simulink model "Acceleration_Angular__Spectrum_Analyser"  (R2014a)
settings: Solver=ode45  StartTime=0.0  StopTime=inf  RelTol=1e-3
undefined symbols (not defined in the file): NULL, serial
libraries: instrumentlib x2
settings Model: Creator=ddtdanilo  LastModifiedBy=ddtdanilo

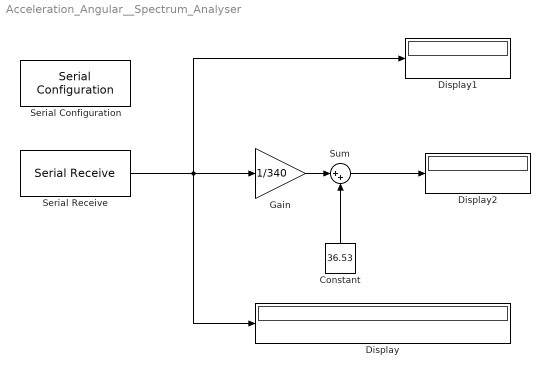
== system Acceleration_Angular__Spectrum_Analyser ==
  Constant : Constant  Value=36.53
  Display : Display
      settings: Format=hex (Stored Integer)
  Display1 : Display
  Display2 : Display
  Gain : Gain  Gain=1/340
  Serial Configuration : instrumentlib/Serial Configuration  Priority=-200000  ComPortMenu=COM7  ComPort=COM7  ObjConstructor=serial('COM7');  BaudRate=115200  DataBits=8  Parity=none  StopBits=1  FlowControl=none  Timeout=2  ByteOrder=LittleEndian
  Serial Receive : instrumentlib/Serial Receive  ComPortMenu=COM7  ComPort=COM7  ObjConstructor=serial('COM7');  Terminator=NULL ('\0')  DataSize="[1  1]"  DataType=int16  EnableBlockingMode=on  ActionDataUnavailable=Error  CustomValue=0  SampleTime=1/100000
  Sum : Sum  Inputs=|++
  wires:
  Serial Receive/1 -> Display1/1, Gain/1, Display/1
  Constant/1 -> Sum/2
  Gain/1 -> Sum/1
  Sum/1 -> Display2/1
